simulink model "cruise_ctrl_old"  (Simulink 8.9)
settings: Solver=FixedStepAuto  StartTime=0.0  StopTime=60  FixedStep=0.01  MaxStep=0.1  RelTol=1e-3  EnableMultiTasking=on
PreLoadFcn:
  | m = 1000;
  | alpha = [40, 25, 16, 12, 10];
  | Tm = 190;
  | wm = 420;
  | beta = 0.4;
  | Cr = 0.01;
  | rho = 1.3;
  | Cd = 0.32;
  | A = 2.4;
  | g = 9.8;
  | theta = 0;
  | gear = 3;
libraries: simulink x1
settings Model: SuppressorTable=22 serialization::archive 11 0 6 0 0 0 11 0  Creator=Cole Lepine  LastModifiedBy=nikhil
settings DataIOCC: SignalLoggingSaveFormat=Dataset
settings OptimizationCC: ExpressionDepthLimit=2147483647  InitFltsAndDblsToZero=on
settings DebuggingCC: SolverPrmCheckMsg=warning
settings GRTTargetCC: GeneratePreprocessorConditionals=Use local settings

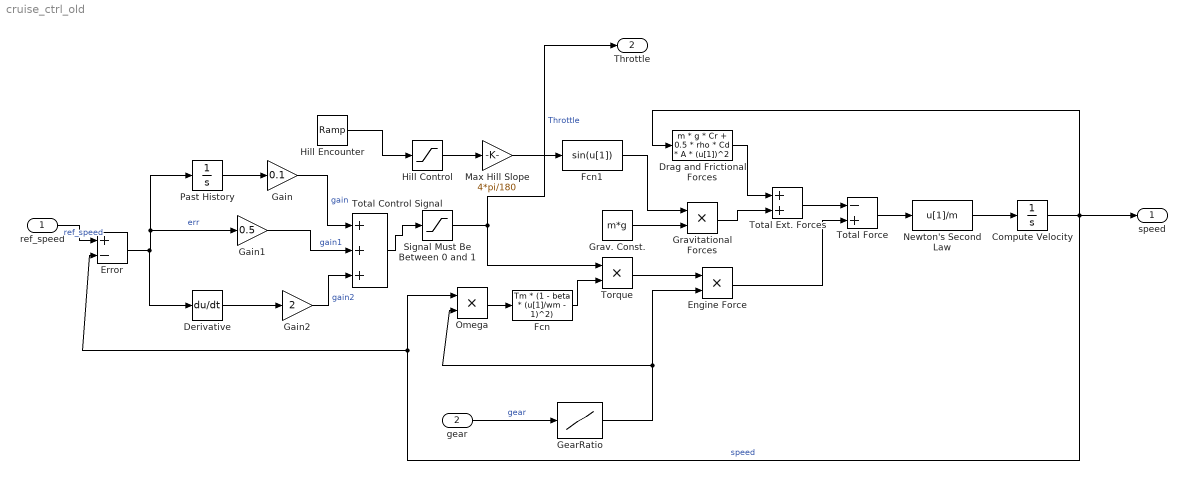
== system cruise_ctrl_old ==
  ref_speed : Inport
  gear : Inport  Port=2
  Compute Velocity : Integrator  InitialCondition=20
  Derivative : Derivative
  Drag and Frictional Forces : Fcn  Expr=m * g * Cr + 0.5 * rho * Cd * A * (u[1])^2
  Engine Force : Product  Inputs=**
  Error : Sum  Inputs=+-
  Fcn : Fcn  Expr=Tm * (1 - beta * (u[1]/wm - 1)^2)
  Fcn1 : Fcn
  Gain : Gain  Gain=0.1
  Gain1 : Gain  Gain=0.5
  Gain2 : Gain  Gain=2
  GearRatio : Lookup_n-D  NumberOfTableDimensions=1  BreakpointsForDimension1=[1,2,3,4,5]  Table=[40,25,16,12,10]  InternalRulePriority=Speed  RndMeth=Simplest  InputSameDT=on
  Grav. Const. : Constant  Value=m*g
  Gravitational Forces : Product  RndMeth=Zero
  Hill Control : Saturate  UpperLimit=1  LowerLimit=0
  Hill Encounter : simulink/Sources/Ramp  slope=1  start=60  X0=0
  Max Hill Slope : Gain  Gain=4*pi/180
  Newton's Second Law : Fcn  Expr=u[1]/m
  Omega : Product  RndMeth=Zero
  Past History : Integrator  InitialCondition=1
  Signal Must Be Between 0 and 1 : Saturate  UpperLimit=1  LowerLimit=0
  Torque : Product  RndMeth=Zero
  Total Ext. Forces : Sum
  Total Control Signal : Sum  Inputs=+++
  Total Force : Sum  Inputs=-+
  speed : Outport
  Throttle : Outport  Port=2
  wires:
  Engine Force/1 -> Total Force/2
  Total Force/1 -> Newton's Second Law/1
  Newton's Second Law/1 -> Compute Velocity/1
  Compute Velocity/1 -> speed/1, Drag and Frictional Forces/1, Omega/1, Error/2  "speed"
  GearRatio/1 -> Engine Force/2, Omega/2
  Omega/1 -> Fcn/1
  Torque/1 -> Engine Force/1
  Fcn/1 -> Torque/2
  Signal Must Be Between 0 and 1/1 -> Throttle/1, Torque/1  "Throttle"
  ref_speed/1 -> Error/1  "ref_speed"
  Total Control Signal/1 -> Signal Must Be Between 0 and 1/1
  Gain1/1 -> Total Control Signal/2  "gain1"
  Gain/1 -> Total Control Signal/1  "gain"
  Past History/1 -> Gain/1
  Total Ext. Forces/1 -> Total Force/1
  Drag and Frictional Forces/1 -> Total Ext. Forces/1
  Gravitational Forces/1 -> Total Ext. Forces/2
  Fcn1/1 -> Gravitational Forces/1
  Max Hill Slope/1 -> Fcn1/1
  Grav. Const./1 -> Gravitational Forces/2
  Hill Control/1 -> Max Hill Slope/1
  Hill Encounter/1 -> Hill Control/1
  Derivative/1 -> Gain2/1
  Error/1 -> Derivative/1, Gain1/1, Past History/1  "err"
  Gain2/1 -> Total Control Signal/3  "gain2"
  gear/1 -> GearRatio/1  "gear"
